simulink model "r_10gbe_demo"  (Simulink 7.0)
settings: Solver=ode45  StartTime=0.0  StopTime=50000  RelTol=1e-3
libraries: xbsIndex_r4 x140, xps_library x42, casper_library x11, xbsReplacements_r4 x3
(part 1 of 2)
settings Model: Creator=dsp  LastModifiedBy=dsp
settings DebuggingCC: SaveWithParameterizedLinksMsg=none  SignalResolutionControl=TryResolveAllWithWarning  MultiTaskDSMMsg=warning  MultiTaskCondExecSysMsg=none  StrictBusMsg=None
settings RTWCC: IncludeERTFirstTime=on
settings GRTTargetCC: TargetFcnLib=ansi_tfl_tmw.mat

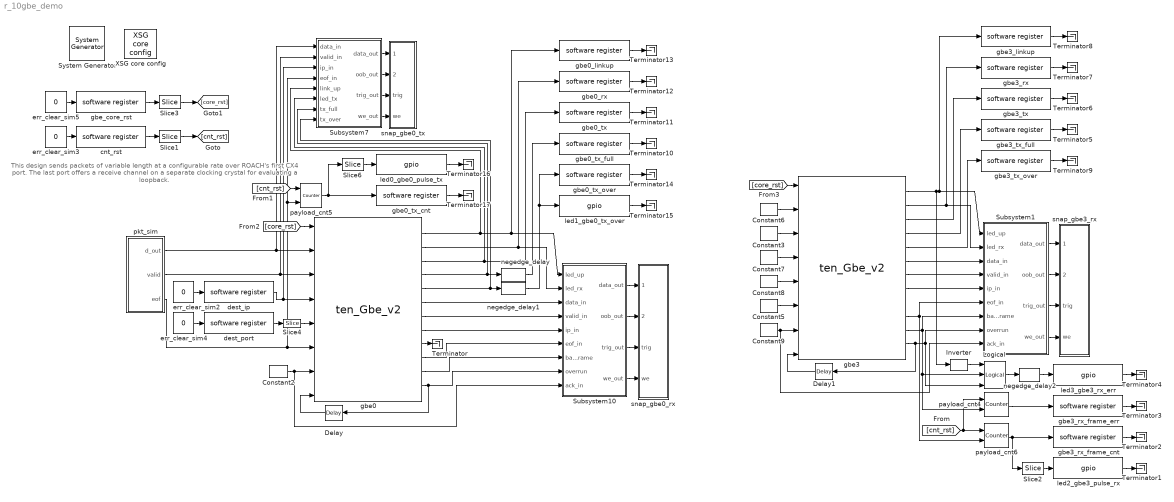
== system r_10gbe_demo ==
  note: This design sends packets of variable length at a configurable rate
      | over ROACH's first CX4 port.
      | The last port offers a receive channel on a separate
      | clocking crystal for evaluating a loopback.
  " System Generator" : xbsIndex_r4/ System Generator  Tag=genX  SystemSampleTime=-1  xilinxfamily=virtex5  part=xc5vsx95t  speed=-1  package=ff1136  synthesis_tool=XST  clock_wrapper=Clock Enables  directory=./r_10gbe_demo/sysgen  testbench=off  simulink_period=1  sysclk_period=5  dcm_input_clock_period=100  incr_netlist=off  trim_vbits=Everywhere in SubSystem  dbl_ovrd=According to Block Masks  core_generation=According to Block Masks  run_coregen=off  deprecated_control=off  eval_field=0  block_type=sysgen
      settings: block_version=10.1.3
  Constant2 : xbsIndex_r4/Constant  arith_type=Boolean  const=1  n_bits=1  bin_pt=0  explicit_period=on  period=1  equ=P=C  opselect=C  inp2=PCIN>>17  opr=+  inp1=P  carry=CIN  dbl_ovrd=off  block_type=constant
  Constant3 : xbsIndex_r4/Constant  arith_type=Boolean  const=0  n_bits=1  bin_pt=0  explicit_period=on  period=1  equ=P=C  opselect=C  inp2=PCIN>>17  opr=+  inp1=P  carry=CIN  dbl_ovrd=off  block_type=constant
  Constant5 : xbsIndex_r4/Constant  arith_type=Boolean  const=0  n_bits=1  bin_pt=0  explicit_period=on  period=1  equ=P=C  opselect=C  inp2=PCIN>>17  opr=+  inp1=P  carry=CIN  dbl_ovrd=off  block_type=constant
  Constant6 : xbsIndex_r4/Constant  arith_type=Unsigned  const=0  n_bits=64  bin_pt=0  explicit_period=on  period=1  equ=P=C  opselect=C  inp2=PCIN>>17  opr=+  inp1=P  carry=CIN  dbl_ovrd=off  block_type=constant
  Constant7 : xbsIndex_r4/Constant  arith_type=Unsigned  const=0  n_bits=32  bin_pt=0  explicit_period=on  period=1  equ=P=C  opselect=C  inp2=PCIN>>17  opr=+  inp1=P  carry=CIN  dbl_ovrd=off  block_type=constant
  Constant8 : xbsIndex_r4/Constant  arith_type=Unsigned  const=0  n_bits=16  bin_pt=0  explicit_period=on  period=1  equ=P=C  opselect=C  inp2=PCIN>>17  opr=+  inp1=P  carry=CIN  dbl_ovrd=off  block_type=constant
  Constant9 : xbsIndex_r4/Constant  arith_type=Boolean  const=1  n_bits=1  bin_pt=0  explicit_period=on  period=1  equ=P=C  opselect=C  inp2=PCIN>>17  opr=+  inp1=P  carry=CIN  dbl_ovrd=off  block_type=constant
  Delay : xbsIndex_r4/Delay  Orientation=left  en=off  latency=1  dbl_ovrd=off  reg_retiming=on  block_type=delay
  Delay1 : xbsIndex_r4/Delay  Orientation=left  en=off  latency=1  dbl_ovrd=off  reg_retiming=on  block_type=delay
  Inverter : xbsIndex_r4/Inverter  en=off  latency=0  dbl_ovrd=off  block_type=inv
  Logical : xbsIndex_r4/Logical  logical_function=OR  inputs=3  en=off  latency=0  precision=Full  arith_type=Unsigned  n_bits=16  bin_pt=0  align_bp=on  dbl_ovrd=off  block_type=logical
  Slice1 : xbsIndex_r4/Slice  nbits=1  boolean_output=on  mode=Lower Bit Location + Width  bit1=0  base1=MSB of Input  bit0=0  base0=LSB of Input  dbl_ovrd=off  block_type=slice
      settings: infoedit="Extracts a given range of bits from each input sample and presents it at the output.  The output type is ordinarily unsigned with binary point at zero, but can be Boolean when the slice is one bit wide.<P><P>Hardware notes: In hardware this block costs nothing."  block_version=10.1.3
  Slice2 : xbsIndex_r4/Slice  nbits=1  boolean_output=on  mode=Lower Bit Location + Width  bit1=0  base1=MSB of Input  bit0=27-12  base0=LSB of Input  dbl_ovrd=off  block_type=slice
      settings: infoedit="Extracts a given range of bits from each input sample and presents it at the output.  The output type is ordinarily unsigned with binary point at zero, but can be Boolean when the slice is one bit wide.<P><P>Hardware notes: In hardware this block costs nothing."  block_version=10.1.3
  Slice3 : xbsIndex_r4/Slice  nbits=1  boolean_output=on  mode=Lower Bit Location + Width  bit1=0  base1=MSB of Input  bit0=0  base0=LSB of Input  dbl_ovrd=off  block_type=slice
      settings: infoedit="Extracts a given range of bits from each input sample and presents it at the output.  The output type is ordinarily unsigned with binary point at zero, but can be Boolean when the slice is one bit wide.<P><P>Hardware notes: In hardware this block costs nothing."  block_version=10.1.3
  Slice4 : xbsIndex_r4/Slice  nbits=16  boolean_output=off  mode=Lower Bit Location + Width  bit1=0  base1=MSB of Input  bit0=0  base0=LSB of Input  dbl_ovrd=off  block_type=slice
      settings: infoedit="Extracts a given range of bits from each input sample and presents it at the output.  The output type is ordinarily unsigned with binary point at zero, but can be Boolean when the slice is one bit wide.<P><P>Hardware notes: In hardware this block costs nothing."  block_version=10.1.3
  Slice6 : xbsIndex_r4/Slice  nbits=1  boolean_output=on  mode=Lower Bit Location + Width  bit1=0  base1=MSB of Input  bit0=27-12  base0=LSB of Input  dbl_ovrd=off  block_type=slice
      settings: infoedit="Extracts a given range of bits from each input sample and presents it at the output.  The output type is ordinarily unsigned with binary point at zero, but can be Boolean when the slice is one bit wide.<P><P>Hardware notes: In hardware this block costs nothing."  block_version=10.1.3
  Subsystem1 : Subsystem
  Subsystem10 : Subsystem
  Subsystem7 : Subsystem
  Terminator{,1..17} (18 alike) : Terminator
  XSG core config : xps_library/XSG core config  Tag=xps:xsg  SystemSampleTime=-1  hw_sys=ROACH:sx95t  ibob_linux=off  clk_src=sys_clk2x  iBOB_clk_src=sys_clk  BEE2_ctrl_clk_src=sys_clk  BEE2_usr_clk_src=sys_clk  ROACH_clk_src=sys_clk2x  CORR_clk_src=sys_clk  gpio_clk_io_group=iBOB:sma  gpio_clk_bit_index=0  clk_rate=200  sample_period=1  synthesis_tool=XST  mpc_type=powerpc440_ext
  cnt_rst : xps_library/software register  Tag=xps:sw_reg  SystemSampleTime=-1  io_dir=From Processor  arith_type=Unsigned  bitwidth=32  bin_pt=0  sample_period=1  gw_name=r_10gbe_demo_cnt_rst_user_data_out
      link override r_10gbe_demo_cnt_rst_user_data_out: arith_type=Unsigned  n_bits=32  bin_pt=0  period=1
      link override r_10gbe_test_cnt_rst_user_data_out: arith_type=Unsigned  n_bits=32  bin_pt=0  period=1
      link override r_xaui_test_cnt_rst_user_data_out: arith_type=Unsigned  n_bits=32  bin_pt=0  period=1
  dest_ip : xps_library/software register  Tag=xps:sw_reg  SystemSampleTime=-1  io_dir=From Processor  arith_type=Unsigned  bitwidth=32  bin_pt=0  sample_period=1  gw_name=r_10gbe_demo_dest_ip_user_data_out
      link override r_10gbe_demo_dest_ip_user_data_out: arith_type=Unsigned  n_bits=32  bin_pt=0  period=1
      link override r_10gbe_test_dest_ip_user_data_out: arith_type=Unsigned  n_bits=32  bin_pt=0  period=1
      link override r_xaui_test_cnt_rst_user_data_out: arith_type=Unsigned  n_bits=32  bin_pt=0  period=1
  dest_port : xps_library/software register  Tag=xps:sw_reg  SystemSampleTime=-1  io_dir=From Processor  arith_type=Unsigned  bitwidth=32  bin_pt=0  sample_period=1  gw_name=r_10gbe_demo_dest_port_user_data_out
      link override r_10gbe_demo_dest_port_user_data_out: arith_type=Unsigned  n_bits=32  bin_pt=0  period=1
      link override r_10gbe_test_dest_port_user_data_out: arith_type=Unsigned  n_bits=32  bin_pt=0  period=1
      link override r_xaui_test_cnt_rst_user_data_out: arith_type=Unsigned  n_bits=32  bin_pt=0  period=1
  err_clear_sim{2..5} (4 alike) : Constant  Value=0  OutDataType=sfix(16)  OutScaling=2^0
  gbe0 : xps_library/ten_Gbe_v2  Tag=xps:tengbe_v2  SystemSampleTime=-1  port=0  rx_dist_ram=off  show_param=off  pre_emph=3  swing=800  fab_en=off  fab_mac=hex2dec('123456780000')  fab_ip=192*(2^24) + 168*(2^16) + 5*(2^8) + 20*(2^0)  fab_udp=10000  fab_gate=1  cpu_rx_en=on  cpu_tx_en=on
  gbe0_linkup : xps_library/software register  Tag=xps:sw_reg  SystemSampleTime=-1  io_dir=To Processor  arith_type=Unsigned  bitwidth=32  bin_pt=0  sample_period=1  gw_name=r_10gbe_demo_gbe0_linkup_user_data_in
      link override convert: arith_type=Unsigned  n_bits=32  bin_pt=0
  gbe0_rx : xps_library/software register  Tag=xps:sw_reg  SystemSampleTime=-1  io_dir=To Processor  arith_type=Unsigned  bitwidth=32  bin_pt=0  sample_period=1  gw_name=r_10gbe_demo_gbe0_rx_user_data_in
      link override convert: arith_type=Unsigned  n_bits=32  bin_pt=0
  gbe0_tx : xps_library/software register  Tag=xps:sw_reg  SystemSampleTime=-1  io_dir=To Processor  arith_type=Unsigned  bitwidth=32  bin_pt=0  sample_period=1  gw_name=r_10gbe_demo_gbe0_tx_user_data_in
      link override convert: arith_type=Unsigned  n_bits=32  bin_pt=0
  gbe0_tx_cnt : xps_library/software register  Tag=xps:sw_reg  SystemSampleTime=-1  io_dir=To Processor  arith_type=Unsigned  bitwidth=32  bin_pt=0  sample_period=1  gw_name=r_10gbe_demo_gbe0_tx_cnt_user_data_in
      link override convert: arith_type=Unsigned  n_bits=32  bin_pt=0
  gbe0_tx_full : xps_library/software register  Tag=xps:sw_reg  SystemSampleTime=-1  io_dir=To Processor  arith_type=Unsigned  bitwidth=32  bin_pt=0  sample_period=1  gw_name=r_10gbe_demo_gbe0_tx_full_user_data_in
      link override convert: arith_type=Unsigned  n_bits=32  bin_pt=0
  gbe0_tx_over : xps_library/software register  Tag=xps:sw_reg  SystemSampleTime=-1  io_dir=To Processor  arith_type=Unsigned  bitwidth=32  bin_pt=0  sample_period=1  gw_name=r_10gbe_demo_gbe0_tx_over_user_data_in
      link override convert: arith_type=Unsigned  n_bits=32  bin_pt=0
  gbe3 : xps_library/ten_Gbe_v2  Tag=xps:tengbe_v2  SystemSampleTime=-1  port=3  rx_dist_ram=off  show_param=off  pre_emph=3  swing=800  fab_en=off  fab_mac=hex2dec('123456780000')  fab_ip=192*(2^24) + 168*(2^16) + 5*(2^8) + 20*(2^0)  fab_udp=10000  fab_gate=1  cpu_rx_en=on  cpu_tx_en=on
  gbe3_linkup : xps_library/software register  Tag=xps:sw_reg  SystemSampleTime=-1  io_dir=To Processor  arith_type=Unsigned  bitwidth=32  bin_pt=0  sample_period=1  gw_name=r_10gbe_demo_gbe3_linkup_user_data_in
      link override convert: arith_type=Unsigned  n_bits=32  bin_pt=0
  gbe3_rx : xps_library/software register  Tag=xps:sw_reg  SystemSampleTime=-1  io_dir=To Processor  arith_type=Unsigned  bitwidth=32  bin_pt=0  sample_period=1  gw_name=r_10gbe_demo_gbe3_rx_user_data_in
      link override convert: arith_type=Unsigned  n_bits=32  bin_pt=0
  gbe3_rx_frame_cnt : xps_library/software register  Tag=xps:sw_reg  SystemSampleTime=-1  io_dir=To Processor  arith_type=Unsigned  bitwidth=32  bin_pt=0  sample_period=1  gw_name=r_10gbe_demo_gbe3_rx_frame_cnt_user_data_in
      link override convert: arith_type=Unsigned  n_bits=32  bin_pt=0
  gbe3_rx_frame_err : xps_library/software register  Tag=xps:sw_reg  SystemSampleTime=-1  io_dir=To Processor  arith_type=Unsigned  bitwidth=32  bin_pt=0  sample_period=1  gw_name=r_10gbe_demo_gbe3_rx_frame_err_user_data_in
      link override convert: arith_type=Unsigned  n_bits=32  bin_pt=0
  gbe3_tx : xps_library/software register  Tag=xps:sw_reg  SystemSampleTime=-1  io_dir=To Processor  arith_type=Unsigned  bitwidth=32  bin_pt=0  sample_period=1  gw_name=r_10gbe_demo_gbe3_tx_user_data_in
      link override convert: arith_type=Unsigned  n_bits=32  bin_pt=0
  gbe3_tx_full : xps_library/software register  Tag=xps:sw_reg  SystemSampleTime=-1  io_dir=To Processor  arith_type=Unsigned  bitwidth=32  bin_pt=0  sample_period=1  gw_name=r_10gbe_demo_gbe3_tx_full_user_data_in
      link override convert: arith_type=Unsigned  n_bits=32  bin_pt=0
  gbe3_tx_over : xps_library/software register  Tag=xps:sw_reg  SystemSampleTime=-1  io_dir=To Processor  arith_type=Unsigned  bitwidth=32  bin_pt=0  sample_period=1  gw_name=r_10gbe_demo_gbe3_tx_over_user_data_in
      link override convert: arith_type=Unsigned  n_bits=32  bin_pt=0
  gbe_core_rst : xps_library/software register  Tag=xps:sw_reg  SystemSampleTime=-1  io_dir=From Processor  arith_type=Unsigned  bitwidth=32  bin_pt=0  sample_period=1  gw_name=r_10gbe_demo_gbe_core_rst_user_data_out
      link override r_10gbe_demo_gbe_core_rst_user_data_out: arith_type=Unsigned  n_bits=32  bin_pt=0  period=1
      link override r_10gbe_test_cnt_rst_user_data_out: arith_type=Unsigned  n_bits=32  bin_pt=0  period=1
      link override r_10gbe_test_gbe_core_rst_user_data_out: arith_type=Unsigned  n_bits=32  bin_pt=0  period=1
      link override r_xaui_test_cnt_rst_user_data_out: arith_type=Unsigned  n_bits=32  bin_pt=0  period=1
  led0_gbe0_pulse_tx : xps_library/gpio  Tag=xps:gpio  SystemSampleTime=-1  io_group=ROACH:led  io_dir=out  arith_type=Boolean  bitwidth=1  bin_pt=0  bit_index=0  sample_period=1  use_single_ended=off  use_ddr=off  reg_iob=off  reg_clk_phase=0  termination=None
      link override convert: arith_type=Boolean  n_bits=1  bin_pt=0
  led1_gbe0_tx_over : xps_library/gpio  Tag=xps:gpio  SystemSampleTime=-1  io_group=ROACH:led  io_dir=out  arith_type=Boolean  bitwidth=1  bin_pt=0  bit_index=1  sample_period=1  use_single_ended=off  use_ddr=off  reg_iob=off  reg_clk_phase=0  termination=None
      link override convert: arith_type=Boolean  n_bits=1  bin_pt=0
  led2_gbe3_pulse_rx : xps_library/gpio  Tag=xps:gpio  SystemSampleTime=-1  io_group=ROACH:led  io_dir=out  arith_type=Boolean  bitwidth=1  bin_pt=0  bit_index=2  sample_period=1  use_single_ended=off  use_ddr=off  reg_iob=off  reg_clk_phase=0  termination=None
      link override convert: arith_type=Boolean  n_bits=1  bin_pt=0
  led3_gbe3_rx_err : xps_library/gpio  Tag=xps:gpio  SystemSampleTime=-1  io_group=ROACH:led  io_dir=out  arith_type=Boolean  bitwidth=1  bin_pt=0  bit_index=3  sample_period=1  use_single_ended=off  use_ddr=off  reg_iob=off  reg_clk_phase=0  termination=None
      link override convert: arith_type=Boolean  n_bits=1  bin_pt=0
  negedge_delay : casper_library/Misc/negedge_delay  SystemSampleTime=-1  pulse_len=2^20
  negedge_delay1 : casper_library/Misc/negedge_delay  SystemSampleTime=-1  pulse_len=2^20
  negedge_delay2 : casper_library/Misc/negedge_delay  SystemSampleTime=-1  pulse_len=2^20
  payload_cnt4 : xbsIndex_r4/Counter  cnt_type=Free Running  cnt_to=0  operation=Up  start_count=0  cnt_by_val=1  arith_type=Unsigned  n_bits=32  bin_pt=0  load_pin=off  rst=on  en=on  explicit_period=on  period=1  dbl_ovrd=off  use_behavioral_HDL=off  use_rpm=on  implementation=Fabric  block_type=counter
      settings: xl_area=[0, 0, 0, 0, 0, 0, 0]
  payload_cnt5 : xbsIndex_r4/Counter  cnt_type=Free Running  cnt_to=0  operation=Up  start_count=0  cnt_by_val=1  arith_type=Unsigned  n_bits=32  bin_pt=0  load_pin=off  rst=on  en=on  explicit_period=on  period=1  dbl_ovrd=off  use_behavioral_HDL=off  use_rpm=on  implementation=Fabric  block_type=counter
      settings: xl_area=[0, 0, 0, 0, 0, 0, 0]
  payload_cnt6 : xbsIndex_r4/Counter  cnt_type=Free Running  cnt_to=0  operation=Up  start_count=0  cnt_by_val=1  arith_type=Unsigned  n_bits=32  bin_pt=0  load_pin=off  rst=on  en=on  explicit_period=on  period=1  dbl_ovrd=off  use_behavioral_HDL=off  use_rpm=on  implementation=Fabric  block_type=counter
      settings: xl_area=[0, 0, 0, 0, 0, 0, 0]
  pkt_sim : Subsystem
  snap_gbe0_rx : Subsystem  AncestorBlock=casper_library/Scopes/snap64  mask(snap64){nsamples=11}
      mask prompts: nsamples "No. of samples(2^?)"
      mask help:
      | The <i>snap</i> block provides a packaged solution to capturing data from
      | the FPGA fabric and making it accessible from the CPU.  The block comes in
      | 2 flavors: <i>snap</i> (which captures to a 32 bit wide Shared BRAM), and
      | <i>snap64</i> (which captures to 2x32 bit wide Shared BRAMs to effect a
      | 64 bit capture).
      mask Help: eval('xlWeb([getenv(''MLIB_ROOT''), ''\casper_library\doc\snap_usage.html''])')
  snap_gbe0_tx : Subsystem  AncestorBlock=casper_library/Scopes/snap64  mask(snap64){nsamples=11}
      mask prompts: nsamples "No. of samples(2^?)"
      mask help:
      | The <i>snap</i> block provides a packaged solution to capturing data from
      | the FPGA fabric and making it accessible from the CPU.  The block comes in
      | 2 flavors: <i>snap</i> (which captures to a 32 bit wide Shared BRAM), and
      | <i>snap64</i> (which captures to 2x32 bit wide Shared BRAMs to effect a
      | 64 bit capture).
      mask Help: eval('xlWeb([getenv(''MLIB_ROOT''), ''\casper_library\doc\snap_usage.html''])')
  snap_gbe3_rx : Subsystem  AncestorBlock=casper_library/Scopes/snap64  mask(snap64){nsamples=11}
      mask prompts: nsamples "No. of samples(2^?)"
      mask help:
      | The <i>snap</i> block provides a packaged solution to capturing data from
      | the FPGA fabric and making it accessible from the CPU.  The block comes in
      | 2 flavors: <i>snap</i> (which captures to a 32 bit wide Shared BRAM), and
      | <i>snap64</i> (which captures to 2x32 bit wide Shared BRAMs to effect a
      | 64 bit capture).
      mask Help: eval('xlWeb([getenv(''MLIB_ROOT''), ''\casper_library\doc\snap_usage.html''])')
  wires:
  [cnt_rst] -> payload_cnt4/1, payload_cnt6/1
  Constant2/1 -> gbe0/7, Subsystem10/9(ack_in)
  Constant6/1 -> gbe3/2
  Constant3/1 -> gbe3/3
  Constant7/1 -> gbe3/4
  Constant8/1 -> gbe3/5
  Subsystem10/1(data_out) -> snap_gbe0_rx/1(data_in)
  Subsystem10/2(oob_out) -> snap_gbe0_rx/2(oob_in)
  Subsystem10/3(trig_out) -> snap_gbe0_rx/3(trig)
  Subsystem10/4(we_out) -> snap_gbe0_rx/4(we)
  gbe0/6 -> Subsystem10/3(data_in)
  gbe0/7 -> Subsystem10/4(valid_in)
  gbe0/8 -> Subsystem10/5(ip_in)
  gbe0/10 -> Subsystem10/6(eof_in)
  err_clear_sim2/1 -> dest_ip/1
  dest_ip/1 -> gbe0/4, Subsystem7/3(ip_in)
  err_clear_sim4/1 -> dest_port/1
  dest_port/1 -> Slice4/1
  Slice4/1 -> gbe0/5
  gbe0/12 -> Subsystem10/8(overrun), Delay/1
  Delay/1 -> gbe0/8
  pkt_sim/2(valid) -> gbe0/3, Subsystem7/2(valid_in)
  Constant5/1 -> gbe3/6
  Constant9/1 -> gbe3/7, Subsystem1/9(ack_in)
  gbe3/12 -> Delay1/1, Subsystem1/8(overrun), Logical/3
  Delay1/1 -> gbe3/8
  gbe0/5 -> negedge_delay1/1, Subsystem7/8(tx_over)
  gbe0/11 -> Subsystem10/7(bad_frame)
  gbe0/1 -> Subsystem10/1(led_up), gbe0_linkup/1, Subsystem7/5(link_up)
  gbe0/2 -> gbe0_rx/1, Subsystem10/2(led_rx)
  gbe0/3 -> gbe0_tx/1, Subsystem7/6(led_tx)
  gbe0/4 -> negedge_delay/1, Subsystem7/7(tx_full)
  gbe3/10 -> payload_cnt6/2, Subsystem1/6(eof_in)
  gbe3/5 -> gbe3_tx_over/1
  gbe3/11 -> Logical/2, payload_cnt4/2, Subsystem1/7(bad_frame)
  gbe3/1 -> Inverter/1, gbe3_linkup/1, Subsystem1/1(led_up)
  gbe3/2 -> gbe3_rx/1, Subsystem1/2(led_rx)
  gbe3/3 -> gbe3_tx/1
  gbe3/4 -> gbe3_tx_full/1
  Logical/1 -> negedge_delay2/1
  Inverter/1 -> Logical/1
  negedge_delay1/1 -> led1_gbe0_tx_over/1, gbe0_tx_over/1
  negedge_delay/1 -> gbe0_tx_full/1
  negedge_delay2/1 -> led3_gbe3_rx_err/1
  payload_cnt4/1 -> gbe3_rx_frame_err/1
  payload_cnt6/1 -> gbe3_rx_frame_cnt/1, Slice2/1
  payload_cnt5/1 -> Slice6/1, gbe0_tx_cnt/1
  Slice6/1 -> led0_gbe0_pulse_tx/1
  Slice2/1 -> led2_gbe3_pulse_rx/1
  Subsystem7/1(data_out) -> snap_gbe0_tx/1(data_in)
  Subsystem7/2(oob_out) -> snap_gbe0_tx/2(oob_in)
  Subsystem7/3(trig_out) -> snap_gbe0_tx/3(trig)
  Subsystem7/4(we_out) -> snap_gbe0_tx/4(we)
  err_clear_sim5/1 -> gbe_core_rst/1
  gbe_core_rst/1 -> Slice3/1
  Subsystem1/1(data_out) -> snap_gbe3_rx/1(data_in)
  Subsystem1/2(oob_out) -> snap_gbe3_rx/2(oob_in)
  Subsystem1/3(trig_out) -> snap_gbe3_rx/3(trig)
  Subsystem1/4(we_out) -> snap_gbe3_rx/4(we)
  gbe3/6 -> Subsystem1/3(data_in)
  gbe3/7 -> Subsystem1/4(valid_in)
  gbe3/8 -> Subsystem1/5(ip_in)
  pkt_sim/1(d_out) -> gbe0/2, Subsystem7/1(data_in)
  pkt_sim/3(eof) -> gbe0/6, payload_cnt5/2, Subsystem7/4(eof_in)
  err_clear_sim3/1 -> cnt_rst/1
  cnt_rst/1 -> Slice1/1
  Slice1/1 -> [cnt_rst]
  [cnt_rst] -> payload_cnt5/1
  Slice3/1 -> [core_rst]
  [core_rst] -> gbe0/1
  [core_rst] -> gbe3/1
  gbe0/9 -> Terminator/1
  led3_gbe3_rx_err/1 -> Terminator4/1
  gbe3_rx_frame_err/1 -> Terminator3/1
  gbe3_rx_frame_cnt/1 -> Terminator2/1
  led2_gbe3_pulse_rx/1 -> Terminator1/1
  gbe3_linkup/1 -> Terminator8/1
  gbe3_rx/1 -> Terminator7/1
  gbe3_tx/1 -> Terminator6/1
  gbe3_tx_full/1 -> Terminator5/1
  gbe3_tx_over/1 -> Terminator9/1
  gbe0_linkup/1 -> Terminator13/1
  gbe0_rx/1 -> Terminator12/1
  gbe0_tx/1 -> Terminator11/1
  gbe0_tx_full/1 -> Terminator10/1
  gbe0_tx_over/1 -> Terminator14/1
  led1_gbe0_tx_over/1 -> Terminator15/1
  led0_gbe0_pulse_tx/1 -> Terminator16/1
  gbe0_tx_cnt/1 -> Terminator17/1

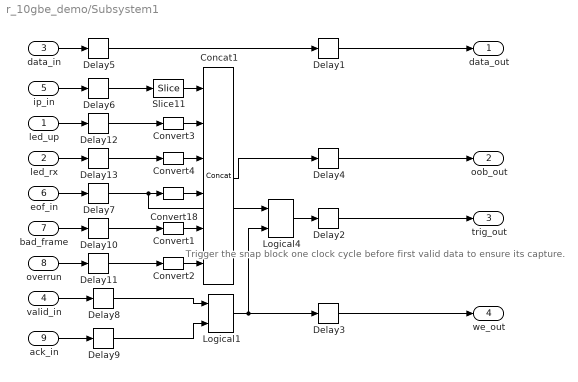
== system r_10gbe_demo/Subsystem1 ==
  note: Trigger the snap block
      | one clock cycle before
      | first valid data to ensure
      | its capture.
  led_up : Inport  OutDataType=sfix(16)  OutScaling=2^0
  led_rx : Inport  Port=2  OutDataType=sfix(16)  OutScaling=2^0
  data_in : Inport  Port=3  OutDataType=sfix(16)  OutScaling=2^0
  valid_in : Inport  Port=4  OutDataType=sfix(16)  OutScaling=2^0
  ip_in : Inport  Port=5  OutDataType=sfix(16)  OutScaling=2^0
  eof_in : Inport  Port=6  OutDataType=sfix(16)  OutScaling=2^0
  bad_frame : Inport  Port=7  OutDataType=sfix(16)  OutScaling=2^0
  overrun : Inport  Port=8  OutDataType=sfix(16)  OutScaling=2^0
  ack_in : Inport  Port=9  OutDataType=sfix(16)  OutScaling=2^0
  Concat1 : xbsIndex_r4/Concat  num_inputs=6  dbl_ovrd=off  block_type=concat
      settings: block_version=10.1.3
  Convert{1..4,18} (5 alike) : xbsIndex_r4/Convert  arith_type=Unsigned  n_bits=1  bin_pt=0  quantization=Truncate  overflow=Wrap  latency=0  dbl_ovrd=off  pipeline=off  block_type=convert
      settings: xl_area=[0, 0, 0, 0, 0, 0, 0]  block_version=10.1.3
  Delay{1..13} (13 alike) : xbsIndex_r4/Delay  en=off  latency=2  dbl_ovrd=off  reg_retiming=on  block_type=delay
      settings: xl_area=[0, 0, 0, 0, 0, 0, 0]
  Logical1 : xbsIndex_r4/Logical  logical_function=AND  inputs=2  en=off  latency=0  precision=Full  arith_type=Unsigned  n_bits=8  bin_pt=2  align_bp=on  dbl_ovrd=off  block_type=logical
      settings: xl_area=[0, 0, 0, 0, 0, 0, 0]
  Logical4 : xbsIndex_r4/Logical  logical_function=AND  inputs=2  en=off  latency=0  precision=Full  arith_type=Unsigned  n_bits=8  bin_pt=2  align_bp=on  dbl_ovrd=off  block_type=logical
      settings: xl_area=[0, 0, 0, 0, 0, 0, 0]
  Slice11 : xbsIndex_r4/Slice  nbits=32-5  boolean_output=off  mode=Lower Bit Location + Width  bit1=0  base1=MSB of Input  bit0=0  base0=LSB of Input  dbl_ovrd=off  block_type=slice
      settings: infoedit="Extracts a given range of bits from each input sample and presents it at the output.  The output type is ordinarily unsigned with binary point at zero, but can be Boolean when the slice is one bit wide.<P><P>Hardware notes: In hardware this block costs nothing."  block_version=10.1.3
  data_out : Outport  OutDataType=sfix(16)  OutScaling=2^0
  oob_out : Outport  Port=2  OutDataType=sfix(16)  OutScaling=2^0
  trig_out : Outport  Port=3  OutDataType=sfix(16)  OutScaling=2^0
  we_out : Outport  Port=4  OutDataType=sfix(16)  OutScaling=2^0
  wires:
  Convert2/1 -> Concat1/6
  Convert1/1 -> Concat1/5
  Convert18/1 -> Concat1/4
  Convert4/1 -> Concat1/3
  Convert3/1 -> Concat1/2
  Slice11/1 -> Concat1/1
  Delay13/1 -> Convert4/1
  led_rx/1 -> Delay13/1
  Delay12/1 -> Convert3/1
  led_up/1 -> Delay12/1
  Delay11/1 -> Convert2/1
  overrun/1 -> Delay11/1
  Delay10/1 -> Convert1/1
  bad_frame/1 -> Delay10/1
  Delay9/1 -> Logical1/2
  Delay8/1 -> Logical1/1
  Delay7/1 -> Convert18/1, Logical4/1
  Delay6/1 -> Slice11/1
  Delay5/1 -> Delay1/1
  Delay3/1 -> we_out/1
  Delay2/1 -> trig_out/1
  Logical1/1 -> Delay3/1, Logical4/2
  ack_in/1 -> Delay9/1
  eof_in/1 -> Delay7/1
  valid_in/1 -> Delay8/1
  Logical4/1 -> Delay2/1
  Delay4/1 -> oob_out/1
  Delay1/1 -> data_out/1
  ip_in/1 -> Delay6/1
  data_in/1 -> Delay5/1
  Concat1/1 -> Delay4/1

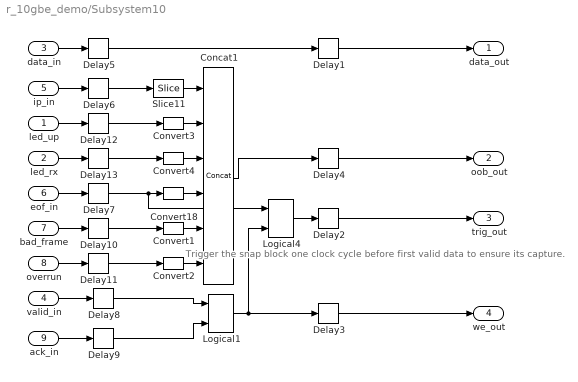
== system r_10gbe_demo/Subsystem10 ==
  note: Trigger the snap block
      | one clock cycle before
      | first valid data to ensure
      | its capture.
  led_up : Inport  OutDataType=sfix(16)  OutScaling=2^0
  led_rx : Inport  Port=2  OutDataType=sfix(16)  OutScaling=2^0
  data_in : Inport  Port=3  OutDataType=sfix(16)  OutScaling=2^0
  valid_in : Inport  Port=4  OutDataType=sfix(16)  OutScaling=2^0
  ip_in : Inport  Port=5  OutDataType=sfix(16)  OutScaling=2^0
  eof_in : Inport  Port=6  OutDataType=sfix(16)  OutScaling=2^0
  bad_frame : Inport  Port=7  OutDataType=sfix(16)  OutScaling=2^0
  overrun : Inport  Port=8  OutDataType=sfix(16)  OutScaling=2^0
  ack_in : Inport  Port=9  OutDataType=sfix(16)  OutScaling=2^0
  Concat1 : xbsIndex_r4/Concat  num_inputs=6  dbl_ovrd=off  block_type=concat
      settings: block_version=10.1.3
  Convert{1..4,18} (5 alike) : xbsIndex_r4/Convert  arith_type=Unsigned  n_bits=1  bin_pt=0  quantization=Truncate  overflow=Wrap  latency=0  dbl_ovrd=off  pipeline=off  block_type=convert
      settings: xl_area=[0, 0, 0, 0, 0, 0, 0]  block_version=10.1.3
  Delay{1..13} (13 alike) : xbsIndex_r4/Delay  en=off  latency=2  dbl_ovrd=off  reg_retiming=on  block_type=delay
      settings: xl_area=[0, 0, 0, 0, 0, 0, 0]
  Logical1 : xbsIndex_r4/Logical  logical_function=AND  inputs=2  en=off  latency=0  precision=Full  arith_type=Unsigned  n_bits=8  bin_pt=2  align_bp=on  dbl_ovrd=off  block_type=logical
      settings: xl_area=[0, 0, 0, 0, 0, 0, 0]
  Logical4 : xbsIndex_r4/Logical  logical_function=AND  inputs=2  en=off  latency=0  precision=Full  arith_type=Unsigned  n_bits=8  bin_pt=2  align_bp=on  dbl_ovrd=off  block_type=logical
      settings: xl_area=[0, 0, 0, 0, 0, 0, 0]
  Slice11 : xbsIndex_r4/Slice  nbits=32-5  boolean_output=off  mode=Lower Bit Location + Width  bit1=0  base1=MSB of Input  bit0=0  base0=LSB of Input  dbl_ovrd=off  block_type=slice
      settings: infoedit="Extracts a given range of bits from each input sample and presents it at the output.  The output type is ordinarily unsigned with binary point at zero, but can be Boolean when the slice is one bit wide.<P><P>Hardware notes: In hardware this block costs nothing."  block_version=10.1.3
  data_out : Outport  OutDataType=sfix(16)  OutScaling=2^0
  oob_out : Outport  Port=2  OutDataType=sfix(16)  OutScaling=2^0
  trig_out : Outport  Port=3  OutDataType=sfix(16)  OutScaling=2^0
  we_out : Outport  Port=4  OutDataType=sfix(16)  OutScaling=2^0
  wires:
  Concat1/1 -> Delay4/1
  data_in/1 -> Delay5/1
  ip_in/1 -> Delay6/1
  Delay1/1 -> data_out/1
  Delay4/1 -> oob_out/1
  Logical4/1 -> Delay2/1
  valid_in/1 -> Delay8/1
  eof_in/1 -> Delay7/1
  ack_in/1 -> Delay9/1
  Logical1/1 -> Logical4/2, Delay3/1
  Delay2/1 -> trig_out/1
  Delay3/1 -> we_out/1
  Delay5/1 -> Delay1/1
  Delay6/1 -> Slice11/1
  Delay7/1 -> Logical4/1, Convert18/1
  Delay8/1 -> Logical1/1
  Delay9/1 -> Logical1/2
  bad_frame/1 -> Delay10/1
  Delay10/1 -> Convert1/1
  overrun/1 -> Delay11/1
  Delay11/1 -> Convert2/1
  led_up/1 -> Delay12/1
  Delay12/1 -> Convert3/1
  led_rx/1 -> Delay13/1
  Delay13/1 -> Convert4/1
  Slice11/1 -> Concat1/1
  Convert3/1 -> Concat1/2
  Convert4/1 -> Concat1/3
  Convert18/1 -> Concat1/4
  Convert1/1 -> Concat1/5
  Convert2/1 -> Concat1/6

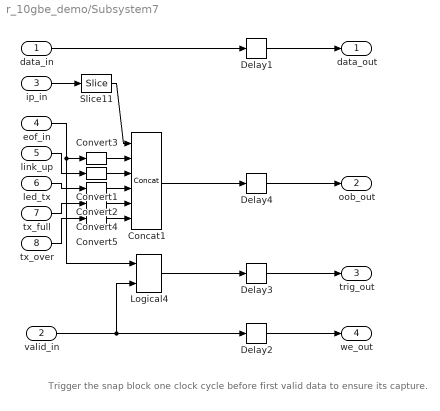
== system r_10gbe_demo/Subsystem7 ==
  note: Trigger the snap block
      | one clock cycle before
      | first valid data to ensure
      | its capture.
  data_in : Inport  OutDataType=sfix(16)  OutScaling=2^0
  valid_in : Inport  Port=2  OutDataType=sfix(16)  OutScaling=2^0
  ip_in : Inport  Port=3  OutDataType=sfix(16)  OutScaling=2^0
  eof_in : Inport  Port=4  OutDataType=sfix(16)  OutScaling=2^0
  link_up : Inport  Port=5  OutDataType=sfix(16)  OutScaling=2^0
  led_tx : Inport  Port=6  OutDataType=sfix(16)  OutScaling=2^0
  tx_full : Inport  Port=7  OutDataType=sfix(16)  OutScaling=2^0
  tx_over : Inport  Port=8  OutDataType=sfix(16)  OutScaling=2^0
  Concat1 : xbsIndex_r4/Concat  num_inputs=6  dbl_ovrd=off  block_type=concat
      settings: block_version=10.1.3
  Convert{1..5} (5 alike) : xbsIndex_r4/Convert  arith_type=Unsigned  n_bits=1  bin_pt=0  quantization=Truncate  overflow=Wrap  latency=0  dbl_ovrd=off  pipeline=off  block_type=convert
      settings: xl_area=[0, 0, 0, 0, 0, 0, 0]  block_version=10.1.3
  Delay{1..4} (4 alike) : xbsIndex_r4/Delay  en=off  latency=2  dbl_ovrd=off  reg_retiming=on  block_type=delay
      settings: xl_area=[0, 0, 0, 0, 0, 0, 0]
  Logical4 : xbsIndex_r4/Logical  logical_function=AND  inputs=2  en=off  latency=0  precision=Full  arith_type=Unsigned  n_bits=8  bin_pt=2  align_bp=on  dbl_ovrd=off  block_type=logical
      settings: xl_area=[0, 0, 0, 0, 0, 0, 0]
  Slice11 : xbsIndex_r4/Slice  nbits=32-5  boolean_output=off  mode=Lower Bit Location + Width  bit1=0  base1=MSB of Input  bit0=0  base0=LSB of Input  dbl_ovrd=off  block_type=slice
      settings: infoedit="Extracts a given range of bits from each input sample and presents it at the output.  The output type is ordinarily unsigned with binary point at zero, but can be Boolean when the slice is one bit wide.<P><P>Hardware notes: In hardware this block costs nothing."  block_version=10.1.3
  data_out : Outport  OutDataType=sfix(16)  OutScaling=2^0
  oob_out : Outport  Port=2  OutDataType=sfix(16)  OutScaling=2^0
  trig_out : Outport  Port=3  OutDataType=sfix(16)  OutScaling=2^0
  we_out : Outport  Port=4  OutDataType=sfix(16)  OutScaling=2^0
  wires:
  Slice11/1 -> Concat1/1
  Concat1/1 -> Delay4/1
  data_in/1 -> Delay1/1
  ip_in/1 -> Slice11/1
  Delay1/1 -> data_out/1
  Delay4/1 -> oob_out/1
  Logical4/1 -> Delay3/1
  valid_in/1 -> Logical4/2, Delay2/1
  Delay2/1 -> we_out/1
  Delay3/1 -> trig_out/1
  eof_in/1 -> Logical4/1, Convert3/1
  link_up/1 -> Convert1/1
  led_tx/1 -> Convert2/1
  tx_full/1 -> Convert4/1
  tx_over/1 -> Convert5/1
  Convert3/1 -> Concat1/2
  Convert1/1 -> Concat1/3
  Convert2/1 -> Concat1/4
  Convert4/1 -> Concat1/5
  Convert5/1 -> Concat1/6

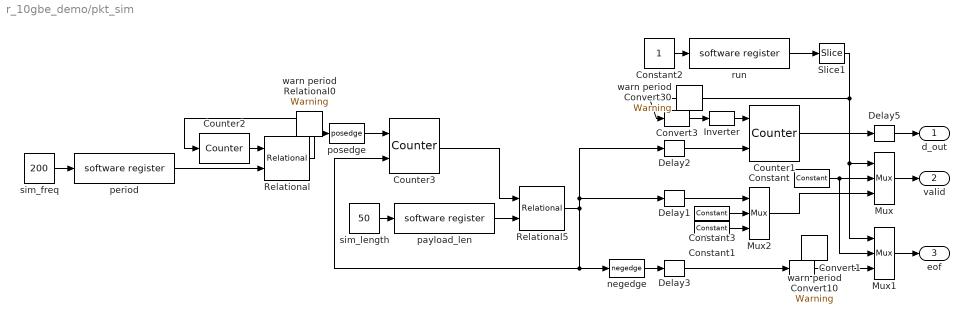
== system r_10gbe_demo/pkt_sim ==
  Constant : xbsIndex_r4/Constant  arith_type=Boolean  const=0  n_bits=1  bin_pt=0  explicit_period=on  period=1  equ=P=C  opselect=C  inp2=PCIN>>17  opr=+  inp1=P  carry=CIN  dbl_ovrd=off  block_type=constant
  Constant1 : xbsIndex_r4/Constant  arith_type=Boolean  const=1  n_bits=1  bin_pt=0  explicit_period=off  period=1  equ=P=C  opselect=C  inp2=PCIN>>17  opr=+  inp1=P  carry=CIN  dbl_ovrd=off  block_type=constant
  Constant2 : Constant  OutDataType=sfix(16)  OutScaling=2^0
  Constant3 : xbsIndex_r4/Constant  arith_type=Boolean  const=0  n_bits=1  bin_pt=0  explicit_period=off  period=1  equ=P=C  opselect=C  inp2=PCIN>>17  opr=+  inp1=P  carry=CIN  dbl_ovrd=off  block_type=constant
  Convert1 : xbsIndex_r4/Convert  arith_type=Boolean  n_bits=8  bin_pt=6  quantization=Truncate  overflow=Wrap  latency=0  dbl_ovrd=off  pipeline=off  block_type=convert
      settings: xl_area=[0, 0, 0, 0, 0, 0, 0]  block_version=10.1.3
  Convert3 : xbsIndex_r4/Convert  arith_type=Boolean  n_bits=8  bin_pt=6  quantization=Truncate  overflow=Wrap  latency=0  dbl_ovrd=off  pipeline=off  block_type=convert
      settings: xl_area=[0, 0, 0, 0, 0, 0, 0]  block_version=10.1.3
  Counter1 : xbsIndex_r4/Counter  cnt_type=Free Running  cnt_to=Inf  operation=Up  start_count=0  cnt_by_val=1  arith_type=Unsigned  n_bits=64  bin_pt=0  load_pin=off  rst=on  en=on  explicit_period=off  period=1  dbl_ovrd=off  use_behavioral_HDL=off  use_rpm=off  implementation=Fabric  block_type=counter
      settings: xl_area=[0, 0, 0, 0, 0, 0, 0]
  Counter2 : xbsIndex_r4/Counter  cnt_type=Free Running  cnt_to=Inf  operation=Up  start_count=1  cnt_by_val=1  arith_type=Unsigned  n_bits=32  bin_pt=0  load_pin=off  rst=on  en=off  explicit_period=on  period=1  dbl_ovrd=off  use_behavioral_HDL=off  use_rpm=on  implementation=Fabric  block_type=counter
      settings: xl_area=[0, 0, 0, 0, 0, 0, 0]
  Counter3 : xbsIndex_r4/Counter  cnt_type=Free Running  cnt_to=1023  operation=Up  start_count=0  cnt_by_val=1  arith_type=Unsigned  n_bits=32  bin_pt=0  load_pin=off  rst=on  en=on  explicit_period=on  period=1  dbl_ovrd=off  use_behavioral_HDL=off  use_rpm=on  implementation=Fabric  block_type=counter
      settings: xl_area=[0, 0, 0, 0, 0, 0, 0]
  Delay{1..3,5} (4 alike) : xbsIndex_r4/Delay  en=off  latency=1  dbl_ovrd=off  reg_retiming=on  block_type=delay
      settings: xl_area=[0, 0, 0, 0, 0, 0, 0]
  Inverter : xbsIndex_r4/Inverter  en=off  latency=0  dbl_ovrd=off  block_type=inv
      settings: xl_area=[0, 0, 0, 0, 0, 0, 0]
  Mux : xbsIndex_r4/Mux  inputs=2  en=off  latency=1  precision=Full  arith_type="Signed  (2's comp)"  n_bits=8  bin_pt=2  quantization=Truncate  overflow=Wrap  dbl_ovrd=off  block_type=mux
      settings: xl_area=[0, 0, 0, 0, 0, 0, 0]
  Mux1 : xbsIndex_r4/Mux  inputs=2  en=off  latency=1  precision=Full  arith_type="Signed  (2's comp)"  n_bits=8  bin_pt=2  quantization=Truncate  overflow=Wrap  dbl_ovrd=off  block_type=mux
      settings: xl_area=[0, 0, 0, 0, 0, 0, 0]
  Mux2 : xbsIndex_r4/Mux  inputs=2  en=off  latency=1  precision=Full  arith_type="Signed  (2's comp)"  n_bits=8  bin_pt=2  quantization=Truncate  overflow=Wrap  dbl_ovrd=off  block_type=mux
      settings: xl_area=[0, 0, 0, 0, 0, 0, 0]
  Relational : xbsIndex_r4/Relational  mode=a>=b  en=off  latency=0  dbl_ovrd=off  block_type=relational
      settings: xl_area=[0, 0, 0, 0, 0, 0, 0]  block_version=10.1.3
  Relational5 : xbsIndex_r4/Relational  mode=a<b  en=off  latency=0  dbl_ovrd=off  block_type=relational
      settings: xl_area=[0, 0, 0, 0, 0, 0, 0]  block_version=10.1.3
  Slice1 : xbsIndex_r4/Slice  nbits=1  boolean_output=off  mode=Lower Bit Location + Width  bit1=1  base1=MSB of Input  bit0=0  base0=LSB of Input  dbl_ovrd=off  block_type=slice
      settings: infoedit="Extracts a given range of bits from each input sample and presents it at the output.  The output type is ordinarily unsigned with binary point at zero, but can be Boolean when the slice is one bit wide.<P><P>Hardware notes: In hardware this block costs nothing."  block_version=10.1.3
  negedge : casper_library/Misc/negedge  Tag=Rising Edge Detector  SystemSampleTime=-1
  payload_len : xps_library/software register  Tag=xps:sw_reg  SystemSampleTime=-1  io_dir=From Processor  arith_type=Unsigned  bitwidth=32  bin_pt=0  sample_period=1  gw_name=r_10gbe_demo_pkt_sim_payload_len_user_data_out
      link override r_10gbe_demo_pkt_sim_payload_len_user_data_out: arith_type=Unsigned  n_bits=32  bin_pt=0  period=1
      link override r_10gbe_test_pkt_sim_payload_len_user_data_out: arith_type=Unsigned  n_bits=32  bin_pt=0  period=1
      link override test_pkt_buffer_10_1_p_mux_up_payload_len_user_data_out: arith_type=Unsigned  n_bits=32  bin_pt=0  period=1
  period : xps_library/software register  Tag=xps:sw_reg  SystemSampleTime=-1  io_dir=From Processor  arith_type=Unsigned  bitwidth=32  bin_pt=0  sample_period=1  gw_name=r_10gbe_demo_pkt_sim_period_user_data_out
      link override r_10gbe_demo_pkt_sim_period_user_data_out: arith_type=Unsigned  n_bits=32  bin_pt=0  period=1
      link override r_10gbe_test_pkt_sim_period_user_data_out: arith_type=Unsigned  n_bits=32  bin_pt=0  period=1
      link override test_pkt_buffer_10_1_p_mux_up_period_user_data_out: arith_type=Unsigned  n_bits=32  bin_pt=0  period=1
  posedge : casper_library/Misc/pulse_ext/posedge  Tag=Rising Edge Detector  SystemSampleTime=-1
  run : xps_library/software register  Tag=xps:sw_reg  SystemSampleTime=-1  io_dir=From Processor  arith_type=Unsigned  bitwidth=32  bin_pt=0  sample_period=1  gw_name=r_10gbe_demo_pkt_sim_run_user_data_out
      link override r_10gbe_demo_pkt_sim_run_user_data_out: arith_type=Unsigned  n_bits=32  bin_pt=0  period=1
      link override r_10gbe_test_pkt_sim_run_user_data_out: arith_type=Unsigned  n_bits=32  bin_pt=0  period=1
      link override test_pkt_buffer_10_1_p_mux_up_run_user_data_out: arith_type=Unsigned  n_bits=32  bin_pt=0  period=1
  sim_freq : Constant  Value=200  OutDataType=sfix(16)  OutScaling=2^0
  sim_length : Constant  Value=50  OutDataType=sfix(16)  OutScaling=2^0
  warn period Convert10 : xbsReplacements_r4/Warning  SystemSampleTime=-1  period=1
  warn period Convert30 : xbsReplacements_r4/Warning  SystemSampleTime=-1  period=1
  warn period Relational0 : xbsReplacements_r4/Warning  SystemSampleTime=-1  period=1
  d_out : Outport  OutDataType=sfix(16)  OutScaling=2^0
  valid : Outport  Port=2  OutDataType=sfix(16)  OutScaling=2^0
  eof : Outport  Port=3  OutDataType=sfix(16)  OutScaling=2^0
  wires:
  Counter2/1 -> Relational/1
  Relational/1 -> posedge/1, Counter2/1
  Counter1/1 -> Delay5/1
  negedge/1 -> Delay3/1
  period/1 -> Relational/2
  sim_freq/1 -> period/1
  Relational5/1 -> Counter3/2, negedge/1, Delay2/1, Delay1/1
  Counter3/1 -> Relational5/1
  posedge/1 -> Counter3/1
  sim_length/1 -> payload_len/1
  payload_len/1 -> Relational5/2
  Mux/1 -> valid/1
  Constant/1 -> Mux/2, Mux1/2
  Mux1/1 -> eof/1
  Delay3/1 -> Convert1/1
  Convert1/1 -> Mux1/3
  Delay5/1 -> d_out/1
  run/1 -> Slice1/1
  Constant2/1 -> run/1
  Slice1/1 -> Mux/1, Mux1/1, Convert3/1
  Mux2/1 -> Mux/3
  Inverter/1 -> Counter1/1
  Delay2/1 -> Counter1/2
  Convert3/1 -> Inverter/1
  Constant3/1 -> Mux2/2
  Constant1/1 -> Mux2/3
  Delay1/1 -> Mux2/1

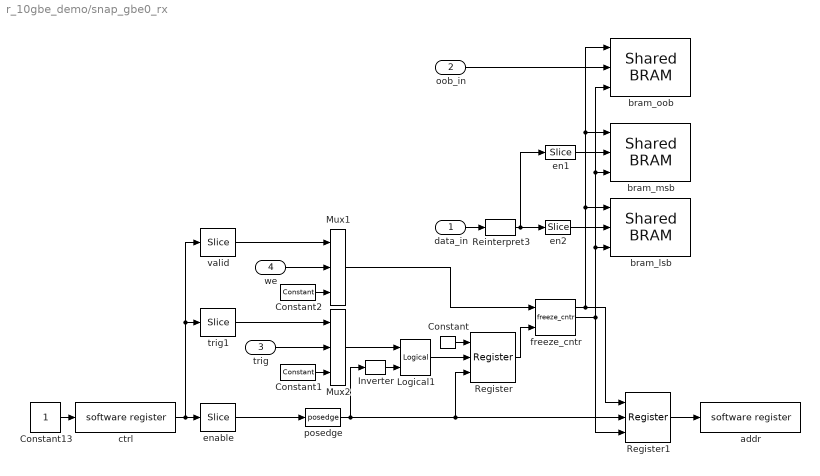
== system r_10gbe_demo/snap_gbe0_rx ==
  data_in : Inport  OutDataType=sfix(16)  OutScaling=2^0
  oob_in : Inport  Port=2  OutDataType=sfix(16)  OutScaling=2^0
  trig : Inport  Port=3  OutDataType=sfix(16)  OutScaling=2^0
  we : Inport  Port=4  OutDataType=sfix(16)  OutScaling=2^0
  Constant : xbsIndex_r4/Constant  arith_type=Boolean  const=1  n_bits=1  bin_pt=0  explicit_period=on  period=1  equ=P=C  opselect=C  inp2=PCIN>>17  opr=+  inp1=P  carry=CIN  dbl_ovrd=off  block_type=constant
  Constant1 : xbsIndex_r4/Constant  arith_type=Boolean  const=1  n_bits=1  bin_pt=0  explicit_period=on  period=1  equ=P=C  opselect=C  inp2=PCIN>>17  opr=+  inp1=P  carry=CIN  dbl_ovrd=off  block_type=constant
  Constant13 : Constant  OutDataType=sfix(16)  OutScaling=2^0
  Constant2 : xbsIndex_r4/Constant  arith_type=Boolean  const=1  n_bits=1  bin_pt=0  explicit_period=on  period=1  equ=P=C  opselect=C  inp2=PCIN>>17  opr=+  inp1=P  carry=CIN  dbl_ovrd=off  block_type=constant
  Inverter : xbsIndex_r4/Inverter  en=off  latency=0  dbl_ovrd=off  block_type=inv
      settings: xl_area=[0, 0, 0, 0, 0, 0, 0]
  Logical1 : xbsIndex_r4/Logical  logical_function=AND  inputs=2  en=off  latency=0  precision=Full  arith_type=Unsigned  n_bits=8  bin_pt=2  align_bp=on  dbl_ovrd=off  block_type=logical
      settings: xl_area=[0, 0, 0, 0, 0, 0, 0]
  Mux1 : xbsIndex_r4/Mux  inputs=2  en=off  latency=0  precision=Full  arith_type="Signed  (2's comp)"  n_bits=8  bin_pt=2  quantization=Truncate  overflow=Wrap  dbl_ovrd=off  block_type=mux
      settings: xl_area=[0, 0, 0, 0, 0, 0, 0]
  Mux2 : xbsIndex_r4/Mux  inputs=2  en=off  latency=0  precision=Full  arith_type="Signed  (2's comp)"  n_bits=8  bin_pt=2  quantization=Truncate  overflow=Wrap  dbl_ovrd=off  block_type=mux
      settings: xl_area=[0, 0, 0, 0, 0, 0, 0]
  Register : xbsIndex_r4/Register  init=0  rst=on  en=on  dbl_ovrd=off  block_type=register
      settings: xl_area=[0, 0, 0, 0, 0, 0, 0]
  Register1 : xbsIndex_r4/Register  init=0  rst=on  en=on  dbl_ovrd=off  block_type=register
      settings: xl_area=[0, 0, 0, 0, 0, 0, 0]
  Reinterpret3 : xbsIndex_r4/Reinterpret  force_arith_type=on  arith_type=Unsigned  force_bin_pt=on  bin_pt=0  block_type=reinterpret
      settings: infoedit="Changes signal type without altering the binary representation.   You can changed the signal between signed and unsigned, and relocate the binary point.<P><P>Hardware notes: In hardware this block costs nothing.<P><P>Example:  Suppose the input is 6 bits wide, signed, with 2 fractional bits, and the output is forced to unsigned with 0 fractional bits.  Then an input of -2.0 (1110.00 in binary 2's complement) becomes an output of 56 (111000 in binary)."  block_version=10.1.3
  addr : xps_library/software register  Tag=xps:sw_reg  SystemSampleTime=-1  io_dir=To Processor  arith_type=Unsigned  bitwidth=32  bin_pt=0  sample_period=1  gw_name=r_10gbe_demo_snap_gbe0_rx_addr_user_data_in
      link override convert: arith_type=Unsigned  n_bits=32  bin_pt=0
  bram_lsb : xps_library/Shared BRAM  Tag=xps:bram  SystemSampleTime=-1  arith_type=Unsigned  addr_width=nsamples  data_width=32  data_bin_pt=0  init_vals=0  sample_rate=1
      link override b_2x_8a_r310b_snap_gbe_rx0_bram_lsb_data_out: arith_type=Unsigned
      link override convert_din: arith_type=Unsigned
      link override mem/sim_data_in: arith_type=Unsigned
      link override r_10gbe_demo_snap_gbe0_rx_bram_lsb_data_out: arith_type=Unsigned
      link override r_10gbe_test_snap_gbe0_rx_bram_lsb_data_out: arith_type=Unsigned
      link override r_2x_8a_r310b_snap_gbe_rx0_bram_lsb_data_out: arith_type=Unsigned
      link override r_2x_8a_r311a_snap_gbe_rx0_bram_lsb_data_out: arith_type=Unsigned
      link override r_2x_8a_r311b_snap_gbe_rx0_bram_lsb_data_out: arith_type=Unsigned
  bram_msb : xps_library/Shared BRAM  Tag=xps:bram  SystemSampleTime=-1  arith_type=Unsigned  addr_width=nsamples  data_width=32  data_bin_pt=0  init_vals=0  sample_rate=1
      link override b_2x_8a_r310b_snap_gbe_rx0_bram_msb_data_out: arith_type=Unsigned
      link override convert_din: arith_type=Unsigned
      link override mem/sim_data_in: arith_type=Unsigned
      link override r_10gbe_demo_snap_gbe0_rx_bram_msb_data_out: arith_type=Unsigned
      link override r_10gbe_test_snap_gbe0_rx_bram_msb_data_out: arith_type=Unsigned
      link override r_2x_8a_r310b_snap_gbe_rx0_bram_msb_data_out: arith_type=Unsigned
      link override r_2x_8a_r311a_snap_gbe_rx0_bram_msb_data_out: arith_type=Unsigned
      link override r_2x_8a_r311b_snap_gbe_rx0_bram_msb_data_out: arith_type=Unsigned
  bram_oob : xps_library/Shared BRAM  Tag=xps:bram  SystemSampleTime=-1  arith_type=Unsigned  addr_width=nsamples  data_width=32  data_bin_pt=0  init_vals=0  sample_rate=1
      link override b_2x_8a_r310b_snap_gbe_rx0_bram_oob_data_out: arith_type=Unsigned
      link override convert_din: arith_type=Unsigned
      link override mem/sim_data_in: arith_type=Unsigned
      link override r_10gbe_demo_snap_gbe0_rx_bram_oob_data_out: arith_type=Unsigned
      link override r_10gbe_test_snap_gbe0_rx_bram_oob_data_out: arith_type=Unsigned
      link override r_2x_8a_r310b_snap_gbe_rx0_bram_oob_data_out: arith_type=Unsigned
      link override r_2x_8a_r311a_snap_gbe_rx0_bram_oob_data_out: arith_type=Unsigned
      link override r_2x_8a_r311b_snap_gbe_rx0_bram_oob_data_out: arith_type=Unsigned
  ctrl : xps_library/software register  Tag=xps:sw_reg  SystemSampleTime=-1  io_dir=From Processor  arith_type=Unsigned  bitwidth=32  bin_pt=0  sample_period=1  gw_name=r_10gbe_demo_snap_gbe0_rx_ctrl_user_data_out
      link override b_2x_8a_r310b_snap_gbe_rx0_ctrl_user_data_out: arith_type=Unsigned  n_bits=32  bin_pt=0  period=1
      link override r_10gbe_demo_snap_gbe0_rx_ctrl_user_data_out: arith_type=Unsigned  n_bits=32  bin_pt=0  period=1
      link override r_10gbe_test_snap_gbe0_rx_ctrl_user_data_out: arith_type=Unsigned  n_bits=32  bin_pt=0  period=1
      link override r_2x_8a_r310b_snap_gbe_rx0_ctrl_user_data_out: arith_type=Unsigned  n_bits=32  bin_pt=0  period=1
      link override r_2x_8a_r311a_snap_gbe_rx0_ctrl_user_data_out: arith_type=Unsigned  n_bits=32  bin_pt=0  period=1
      link override r_2x_8a_r311b_snap_gbe_rx0_ctrl_user_data_out: arith_type=Unsigned  n_bits=32  bin_pt=0  period=1
  en1 : xbsIndex_r4/Slice  nbits=32  boolean_output=off  mode=Lower Bit Location + Width  bit1=0  base1=LSB of Input  bit0=32  base0=LSB of Input  dbl_ovrd=off  block_type=slice
      settings: infoedit="Extracts a given range of bits from each input sample and presents it at the output.  The output type is ordinarily unsigned with binary point at zero, but can be Boolean when the slice is one bit wide.<P><P>Hardware notes: In hardware this block costs nothing."  block_version=10.1.3
  en2 : xbsIndex_r4/Slice  nbits=32  boolean_output=off  mode=Lower Bit Location + Width  bit1=0  base1=LSB of Input  bit0=0  base0=LSB of Input  dbl_ovrd=off  block_type=slice
      settings: infoedit="Extracts a given range of bits from each input sample and presents it at the output.  The output type is ordinarily unsigned with binary point at zero, but can be Boolean when the slice is one bit wide.<P><P>Hardware notes: In hardware this block costs nothing."  block_version=10.1.3
  enable : xbsIndex_r4/Slice  nbits=1  boolean_output=on  mode=Lower Bit Location + Width  bit1=0  base1=LSB of Input  bit0=0  base0=LSB of Input  dbl_ovrd=off  block_type=slice
      settings: infoedit="Extracts a given range of bits from each input sample and presents it at the output.  The output type is ordinarily unsigned with binary point at zero, but can be Boolean when the slice is one bit wide.<P><P>Hardware notes: In hardware this block costs nothing."  block_version=10.1.3
  freeze_cntr : casper_library/Misc/freeze_cntr  SystemSampleTime=-1  CounterBits=nsamples
  posedge : casper_library/Misc/posedge  Tag=Rising Edge Detector  SystemSampleTime=-1
  trig1 : xbsIndex_r4/Slice  nbits=1  boolean_output=on  mode=Lower Bit Location + Width  bit1=0  base1=LSB of Input  bit0=1  base0=LSB of Input  dbl_ovrd=off  block_type=slice
      settings: infoedit="Extracts a given range of bits from each input sample and presents it at the output.  The output type is ordinarily unsigned with binary point at zero, but can be Boolean when the slice is one bit wide.<P><P>Hardware notes: In hardware this block costs nothing."  block_version=10.1.3
  valid : xbsIndex_r4/Slice  nbits=1  boolean_output=on  mode=Lower Bit Location + Width  bit1=0  base1=LSB of Input  bit0=2  base0=LSB of Input  dbl_ovrd=off  block_type=slice
      settings: infoedit="Extracts a given range of bits from each input sample and presents it at the output.  The output type is ordinarily unsigned with binary point at zero, but can be Boolean when the slice is one bit wide.<P><P>Hardware notes: In hardware this block costs nothing."  block_version=10.1.3
  wires:
  freeze_cntr/1 -> bram_lsb/1, bram_msb/1, bram_oob/1, Register1/1
  Register/1 -> freeze_cntr/2
  Mux2/1 -> Logical1/1
  Inverter/1 -> Logical1/2
  Logical1/1 -> Register/2
  valid/1 -> Mux1/1
  trig1/1 -> Mux2/1
  Register1/1 -> addr/1
  Constant2/1 -> Mux1/3
  we/1 -> Mux1/2
  Mux1/1 -> freeze_cntr/1
  Constant1/1 -> Mux2/3
  Constant/1 -> Register/1
  posedge/1 -> Inverter/1, Register1/2, Register/3
  ctrl/1 -> trig1/1, valid/1, enable/1
  Constant13/1 -> ctrl/1
  freeze_cntr/2 -> bram_lsb/3, bram_msb/3, bram_oob/3, Register1/3
  enable/1 -> posedge/1
  trig/1 -> Mux2/2
  Reinterpret3/1 -> en1/1, en2/1
  data_in/1 -> Reinterpret3/1
  en1/1 -> bram_msb/2
  en2/1 -> bram_lsb/2
  oob_in/1 -> bram_oob/2
